simulink library "MOST_Lib"  (R2020b)
settings: Solver=VariableStepAuto  StartTime=0.0  StopTime=10.0  RelTol=1e-3
undefined symbols (not defined in the file): simu, wind, windTurbine, windturbine, X, Y, Z
libraries: nesl_utility x54, sm_lib x50, simulink x4, simulink_extras x1, pid_lib x1, WECSim_Lib_Body_Elements x1
(part 3 of 3)

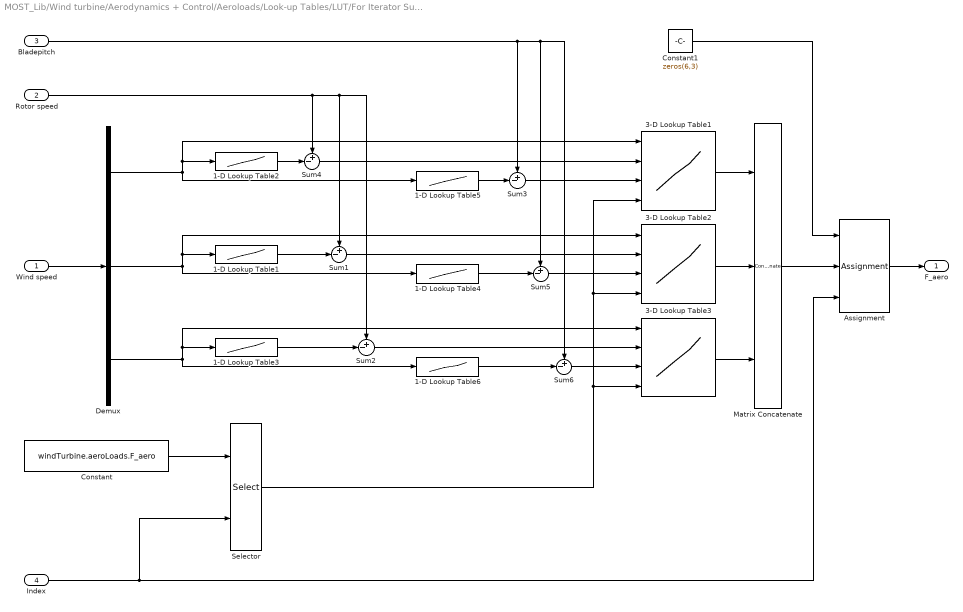
== system MOST_Lib/Wind turbine/Aerodynamics + Control/Aeroloads/Look-up Tables/LUT/For Iterator Subsystem/  ==
  Wind speed : Inport
  Rotor speed : Inport  Port=2
  Bladepitch : Inport  Port=3
  Index : Inport  Port=4
  1-D Lookup Table1 : Lookup_n-D  NumberOfTableDimensions=1  BreakpointsForDimension1=windTurbine.aeroLoads.wind_vec  Table=windTurbine.aeroLoads.omega_vec  InternalRulePriority=Speed  RndMeth=Simplest  InputSameDT=on
  1-D Lookup Table2 : Lookup_n-D  NumberOfTableDimensions=1  BreakpointsForDimension1=windTurbine.aeroLoads.wind_vec  Table=windTurbine.aeroLoads.omega_vec  InternalRulePriority=Speed  RndMeth=Simplest  InputSameDT=on
  1-D Lookup Table3 : Lookup_n-D  NumberOfTableDimensions=1  BreakpointsForDimension1=windTurbine.aeroLoads.wind_vec  Table=windTurbine.aeroLoads.omega_vec  InternalRulePriority=Speed  RndMeth=Simplest  InputSameDT=on
  1-D Lookup Table4 : Lookup_n-D  NumberOfTableDimensions=1  BreakpointsForDimension1=windTurbine.aeroLoads.wind_vec  Table=windTurbine.aeroLoads.bladepitch_vec  InternalRulePriority=Speed  RndMeth=Simplest  InputSameDT=on
  1-D Lookup Table5 : Lookup_n-D  NumberOfTableDimensions=1  BreakpointsForDimension1=windTurbine.aeroLoads.wind_vec  Table=windTurbine.aeroLoads.bladepitch_vec  InternalRulePriority=Speed  RndMeth=Simplest  InputSameDT=on
  1-D Lookup Table6 : Lookup_n-D  NumberOfTableDimensions=1  BreakpointsForDimension1=windTurbine.aeroLoads.wind_vec  Table=windTurbine.aeroLoads.bladepitch_vec  InternalRulePriority=Speed  RndMeth=Simplest  InputSameDT=on
  3-D Lookup Table1 : Lookup_n-D  NumberOfTableDimensions=3  BreakpointsForDimension1=windTurbine.aeroLoads.wind_vec  BreakpointsForDimension2=windTurbine.aeroLoads.omegaerr  BreakpointsForDimension3=windTurbine.aeroLoads.bladepitcherr  TableSource=Input port  Table=squeeze(windturbine.aeroloads.F_aero(:,:,:,1))  ExtrapMethod=Clip  UseLastTableValue=on  InternalRulePriority=Speed  RndMeth=Simplest  InputSameDT=on
      settings: InputPortMap=u0,u1,u2,p221
  3-D Lookup Table2 : Lookup_n-D  NumberOfTableDimensions=3  BreakpointsForDimension1=windTurbine.aeroLoads.wind_vec  BreakpointsForDimension2=windTurbine.aeroLoads.omegaerr  BreakpointsForDimension3=windTurbine.aeroLoads.bladepitcherr  TableSource=Input port  Table=squeeze(windturbine.aeroloads.F_aero(:,:,:,1))  ExtrapMethod=Clip  UseLastTableValue=on  InternalRulePriority=Speed  RndMeth=Simplest  InputSameDT=on
      settings: InputPortMap=u0,u1,u2,p221
  3-D Lookup Table3 : Lookup_n-D  NumberOfTableDimensions=3  BreakpointsForDimension1=windTurbine.aeroLoads.wind_vec  BreakpointsForDimension2=windTurbine.aeroLoads.omegaerr  BreakpointsForDimension3=windTurbine.aeroLoads.bladepitcherr  TableSource=Input port  Table=squeeze(windturbine.aeroloads.F_aero(:,:,:,1))  ExtrapMethod=Clip  UseLastTableValue=on  InternalRulePriority=Speed  RndMeth=Simplest  InputSameDT=on
      settings: InputPortMap=u0,u1,u2,p221
  Assignment : Assignment  NumberOfDimensions=2  DiagnosticForDimensions=Warning  IndexOptions=Index vector (port),Assign all  Indices=1,1  OutputSizes=1,1
  Constant : Constant  Value=windTurbine.aeroLoads.F_aero
  Constant1 : Constant  Value=zeros(6,3)
  Demux : Demux  Outputs=3
  Matrix Concatenate : Concatenate  NumInputs=3  Mode=Multidimensional array  ConcatenateDimension=2
  Selector : Selector  NumberOfDimensions=4  InputPortWidth=3  IndexOptions=Select all,Select all,Select all,Index vector (port)  Indices=[1 3],1,1,1  OutputSizes=1,1,1,1
  Sum{1..6} (6 alike) : Sum  Inputs=+-|
  F_aero : Outport  PortDimensions=[6 3]
  wires:
  Wind speed/1 -> Demux/1
  Demux/3 -> 1-D Lookup Table6/1, 3-D Lookup Table3/1, 1-D Lookup Table3/1
  Demux/2 -> 1-D Lookup Table4/1, 3-D Lookup Table2/1, 1-D Lookup Table1/1
  1-D Lookup Table4/1 -> Sum5/2
  1-D Lookup Table5/1 -> Sum3/2
  1-D Lookup Table6/1 -> Sum6/2
  Sum6/1 -> 3-D Lookup Table3/3
  Sum4/1 -> 3-D Lookup Table1/2
  Sum3/1 -> 3-D Lookup Table1/3
  Demux/1 -> 1-D Lookup Table5/1, 1-D Lookup Table2/1, 3-D Lookup Table1/1
  Sum5/1 -> 3-D Lookup Table2/3
  Sum1/1 -> 3-D Lookup Table2/2
  Sum2/1 -> 3-D Lookup Table3/2
  Rotor speed/1 -> Sum4/1, Sum2/1, Sum1/1
  Constant/1 -> Selector/1
  Index/1 -> Selector/2, Assignment/3
  Selector/1 -> 3-D Lookup Table3/4, 3-D Lookup Table2/4, 3-D Lookup Table1/4
  1-D Lookup Table2/1 -> Sum4/2
  1-D Lookup Table1/1 -> Sum1/2
  1-D Lookup Table3/1 -> Sum2/2
  Bladepitch/1 -> Sum3/1, Sum6/1, Sum5/1
  Assignment/1 -> F_aero/1
  Constant1/1 -> Assignment/1
  3-D Lookup Table1/1 -> Matrix Concatenate/1
  3-D Lookup Table2/1 -> Matrix Concatenate/2
  3-D Lookup Table3/1 -> Matrix Concatenate/3
  Matrix Concatenate/1 -> Assignment/2

== system MOST_Lib/Wind turbine/Aerodynamics + Control/Control/ROSCO/ROSCO controller /Bladepitch control/Integrator with dynamic saturation ==
  omega error : Inport
  minimum pitch : Inport  Port=2
  Constant : Constant  Value=deg2rad(90)
  Gain : Gain  Gain=simu.dt
  Saturation Dynamic : simulink/Discontinuities/Saturation Dynamic  OutMin=[]  OutMax=[]  OutDataTypeStr=Inherit: Same as second input  OutDataType=fixdt(1, 16)  OutScaling=2^-10  DoSatur=off
  Sum : Sum  Inputs=|++
  Unit Delay : UnitDelay  SampleTime=-1  HasFrameUpgradeWarning=on
  integration : Outport
  wires:
  minimum pitch/1 -> Saturation Dynamic/3
  Gain/1 -> Sum/1
  Unit Delay/1 -> Sum/2
  Sum/1 -> Saturation Dynamic/2
  omega error/1 -> Gain/1
  Constant/1 -> Saturation Dynamic/1
  Saturation Dynamic/1 -> Unit Delay/1, integration/1

== matlab function MOST_Lib/Wind turbine/Aerodynamics + Control/Aeroloads/BEM/BEM ==
  data: wind input size=wind.Input.signals.dimensions; q input size=[14 1]; bladepitch input size=1; F_aero_r_bl output size=[6 3]; BEMstruct parameter
function F_aero_r_bl = BEM(wind,q,bladepitch,BEMstruct)

%% INFO

% q: 1-12  -Hub states (no tilt)
%    13    -azimuth
%    14    -rotor omega 

%% CALC AEROLOADS

    pntm=[0 0 0].*BEMstruct.bladedata_r;  
    Cn=0;   Ct=0;    CM=0;
    F_aero_r_bl=zeros(6,3);

           
    R_02hu=Rx(q(4))*Ry(q(5))*Rz(q(6))*BEMstruct.WT_Ry_tilt;
    w_rot_0=q(10:12)+R_02hu*[q(14);0;0];
       
            
    for bl=1:3
        
        R_02bl_root=R_02hu*[1              0                             0             ;
                            0   cos(q(13)+2*pi/3*(bl-1))     -sin(q(13)+2*pi/3*(bl-1)) ;
                            0   sin(q(13)+2*pi/3*(bl-1))      cos(q(13)+2*pi/3*(bl-1))]*BEMstruct.WT_Ry_precone;
        
        a=0;
        at=0;                                                       

        for node=1:length(BEMstruct.bladedata_r)

            
            R_02bl_node=R_02bl_root*[cos(BEMstruct.bladedata_BlCrvAng(node))   0   sin(BEMstruct.bladedata_BlCrvAng(node)) ;
                                                       0                  1                 0                    ;
                                     -sin(BEMstruct.bladedata_BlCrvAng(node))  0   cos(BEMstruct.bladedata_BlCrvAng(node))];


            r_node_0=q(1:3)+R_02bl_root*[BEMstruct.bladedata_BlCrvAC(node);BEMstruct.bladedata_BlSwpAC(node);BEMstruct.bladedata_r(node)];
            v_node_0=q(7:9)+cross(w_rot_0,r_node_0-q(1:3));
           
         
            v_wind_inf_0=[interp3(BEMstruct.WIND_Ydiscr,BEMstruct.WIND_Xdiscr,BEMstruct.WIND_Zdiscr,wind(:,:,:,1),r_node_0(2),r_node_0(1),r_node_0(3));
                          interp3(BEMstruct.WIND_Ydiscr,BEMstruct.WIND_Xdiscr,BEMstruct.WIND_Zdiscr,wind(:,:,:,2),r_node_0(2),r_node_0(1),r_node_0(3));
                          interp3(BEMstruct.WIND_Ydiscr,BEMstruct.WIND_Xdiscr,BEMstruct.WIND_Zdiscr,wind(:,:,:,3),r_node_0(2),r_node_0(1),r_node_0(3))];

            v_wind_rel_bl=R_02bl_node'*(v_wind_inf_0-v_node_0);

            
            VXoverVY=v_wind_rel_bl(1)/v_wind_rel_bl(2);
            s=3*BEMstruct.bladedata_chord(node)/2/pi/BEMstruct.bladedata_r(node);  
            i=1;
            eps=1;

            while eps>BEMstruct.root_tol_rel  &&  i<=BEMstruct.maxit
                phi_i=atan((1-a)/(1+at)*VXoverVY);
                alfa=rad2deg(phi_i-bladepitch)-BEMstruct.bladedata_twist(node);

                CL=interp1(BEMstruct.bladedata_airfoil(:,1,BEMstruct.bladedata_airfoil_index(node)),BEMstruct.bladedata_airfoil(:,2,BEMstruct.bladedata_airfoil_index(node)),alfa);
                CD=interp1(BEMstruct.bladedata_airfoil(:,1,BEMstruct.bladedata_airfoil_index(node)),BEMstruct.bladedata_airfoil(:,3,BEMstruct.bladedata_airfoil_index(node)),alfa);
                CM=interp1(BEMstruct.bladedata_airfoil(:,1,BEMstruct.bladedata_airfoil_index(node)),BEMstruct.bladedata_airfoil(:,4,BEMstruct.bladedata_airfoil_index(node)),alfa);
                Cn=CL*cos(phi_i)+CD*sin(phi_i);
                Ct=CL*sin(phi_i)-CD*cos(phi_i);
               
                Ftip=2/pi*acos(exp(-1.5*(BEMstruct.bladedata_RhubRblade(2)-BEMstruct.bladedata_r(node))/BEMstruct.bladedata_r(node)/abs(sin(phi_i+1e-5)))); % loss tip
                Fhub=2/pi*acos(exp(-1.5*(BEMstruct.bladedata_r(node)-BEMstruct.bladedata_RhubRblade(1))/BEMstruct.bladedata_r(node)/abs(sin(phi_i+1e-5)))); % loss hub
                F=Ftip*Fhub;
               
                k=s*Cn/4/F/sin(phi_i)^2;
                kt=s*Ct/4/F/sin(phi_i)/cos(phi_i);
                if (phi_i>0 && k<=2/3)                
                    a=k/(1+k);                         

                elseif (phi_i>0 && k>2/3)              
                    g1=2*F*k-(10/9-F);
                    g2=2*F*k-F*(4/3-F);
                    g3=2*F*k-(25/9-2*F);
                    a=(g1-sqrt(g2))/g3;                

                elseif (phi_i<0 && k>1)                
                    a=k/(k-1);
                
                elseif (k<=1 && phi_i<0)              
                    a=0;
                end
                
                at=kt/(1-kt);                          

                phi_f=atan((1-a)/(1+at)*VXoverVY);
                i=i+1;
                eps=abs((phi_i-phi_f)/phi_i);

                                
            end
           
           
            if i>BEMstruct.maxit || a==0

                if R(BEMstruct.eps,v_wind_rel_bl(1),bladepitch,q(14),s,node,BEMstruct)*R(pi/2-BEMstruct.eps,v_wind_rel_bl(1),bladepitch,q(14),s,node,BEMstruct)<0
                    phi=Root_find(@(phi)R(phi,v_wind_rel_bl(1),bladepitch,q(14),s,node,BEMstruct),[BEMstruct.eps pi/2],BEMstruct);
                
                elseif Rpb(-pi/4,v_wind_rel_bl(1),bladepitch,q(14),s,node,BEMstruct)*Rpb(-BEMstruct.eps,v_wind_rel_bl(1),bladepitch,q(14),s,node,BEMstruct)<0
                    phi=Root_find(@(phi)Rpb(phi,v_wind_rel_bl(1),bladepitch,q(14),s,node,BEMstruct),[-pi/4 -BEMstruct.eps],BEMstruct);

                else
                    phi=Root_find(@(phi)R(phi,v_wind_rel_bl(1),bladepitch,q(14),s,node,BEMstruct),[pi/2+BEMstruct.eps pi-BEMstruct.eps],BEMstruct);

                end

            alfa=rad2deg(phi-bladepitch)-BEMstruct.bladedata_twist(node);            
            CL=interp1(BEMstruct.bladedata_airfoil(:,1,BEMstruct.bladedata_airfoil_index(node)),BEMstruct.bladedata_airfoil(:,2,BEMstruct.bladedata_airfoil_index(node)),alfa);
            CD=interp1(BEMstruct.bladedata_airfoil(:,1,BEMstruct.bladedata_airfoil_index(node)),BEMstruct.bladedata_airfoil(:,3,BEMstruct.bladedata_airfoil_index(node)),alfa);
            CM=interp1(BEMstruct.bladedata_airfoil(:,1,BEMstruct.bladedata_airfoil_index(node)),BEMstruct.bladedata_airfoil(:,4,BEMstruct.bladedata_airfoil_index(node)),alfa);
            Cn=CL*cos(phi)+CD*sin(phi);
            Ct=CL*sin(phi)-CD*cos(phi);
            Ftip=2/pi*acos(exp(-1.5*(BEMstruct.bladedata_RhubRblade(2)-BEMstruct.bladedata_r(node))/BEMstruct.bladedata_r(node)/abs(sin(phi+1e-5))));
            Fhub=2/pi*acos(exp(-1.5*(BEMstruct.bladedata_r(node)-BEMstruct.bladedata_RhubRblade(1))/BEMstruct.bladedata_r(node)/abs(sin(phi+1e-5))));
            F=Ftip*Fhub;

            kt=s*Ct/4/F/sin(phi)/cos(phi);
            at=kt/(1-kt);
            Vrel2=(v_wind_rel_bl(2)*(1+at)/cos(phi))^2;

            else
            
            Vrel2=(v_wind_rel_bl(1)*(1-a))^2+(v_wind_rel_bl(2)*(1+at))^2;
            
            end
            pntm(node,:)=0.5*BEMstruct.rho_air*BEMstruct.bladedata_chord(node)*Vrel2*[Cn,Ct,CM*BEMstruct.bladedata_chord(node)];        
            

            if anynan([a at])
                a=0; at=0;
            end

        end

        % Remove NaN

        if anynan(pntm)

            temp_y=[[0 0 0];pntm;[0 0 0]];
            temp_x=(1:size(temp_y,1))';
            temp_y=[interp1(temp_x(~isnan(temp_y(:,1))),temp_y(~isnan(temp_y(:,1)),1),temp_x,'linear'),...
                    interp1(temp_x(~isnan(temp_y(:,2))),temp_y(~isnan(temp_y(:,2)),2),temp_x,'linear'),...
                    interp1(temp_x(~isnan(temp_y(:,3))),temp_y(~isnan(temp_y(:,3)),3),temp_x,'linear')];
            pntm=temp_y(2:end-1,:);

        end

        

        F_aero_r_bl(:,bl)=[ (BEMstruct.bladedata_r_int*(pntm(:,1).*cos(BEMstruct.bladedata_BlCrvAng)));
                           -(BEMstruct.bladedata_r_int*pntm(:,2));
                            (BEMstruct.bladedata_r_int*(pntm(:,1).*sin(-BEMstruct.bladedata_BlCrvAng)));
                            (BEMstruct.bladedata_r_int*(pntm(:,2).*(BEMstruct.bladedata_r-BEMstruct.bladedata_RhubRblade(1))*BEMstruct.WT_cos_precone+pntm(:,3).*sin(BEMstruct.bladedata_BlCrvAng)+pntm(:,1).*sin(-BEMstruct.bladedata_BlCrvAng).*BEMstruct.bladedata_BlSwpAC));
                            (BEMstruct.bladedata_r_int*(pntm(:,1).*(BEMstruct.bladedata_r-BEMstruct.bladedata_RhubRblade(1))));
                            (BEMstruct.bladedata_r_int*(pntm(:,3).*cos(BEMstruct.bladedata_BlCrvAng)-pntm(:,1).*cos(BEMstruct.bladedata_BlCrvAng).*BEMstruct.bladedata_BlSwpAC-pntm(:,2).*BEMstruct.bladedata_BlCrvAC))];

        
    end

    

end

%% FUNC

function [root] = Root_find(Fun,Int,BEMstruct)

a = Int(1,1);
b = Int(1,2);
fa = Fun(a);
fb = Fun(b);
it = 0;
s=b;

while abs((b-a)/a)>BEMstruct.root_tol_rel2  &&  it<BEMstruct.maxit2  &&  abs(fb)>BEMstruct.func_tol2

    it = it + 1;
    s = (a + b)/2;
    fs = Fun(s);

    if fa*fs < 0
        b = s;
        fb = fs;
    else
        a = s;
        fa = fs;
    end

end

root = s;

end

% function [root] = Root_find(Fun,Int,ALCS)
% 
% a = Int(1,1);
% b = Int(1,2);
% fa = Fun(a);
% fb = Fun(b);
% fs=fb;
% it = 0;
%                                      
% s=b; c=a;  d=a;    
% mflag = 1;                                
% while abs(b-a)>ALCS.root_tol_rel2 && it<ALCS.maxit2 && abs(fs)>ALCS.func_tol2
%     fc = Fun(c);
%     if fa ~= fc && fb ~=fc                 % inverse quadratic interpolation
%         s = a*fb*fc/((fa - fb)*(fa - fc)) + b*fa*fc/((fb - fa)*(fb - fc))...
%             + c*fa*fb/((fc - fa)*(fc - fb));
%     else                                   % linear interpolation (Secant Method)
%         s = b - fb*(b - a)/(fb - fa);
%     end
%     if (s < min([(3*a + b)/4,b]) || s > max([(3*a + b)/4,b])) || ...
%             (mflag == 1 && abs(s - b) >= abs(b - c)/2) || ...
%             (mflag == 0 && abs(s - b) >= abs(c - d)/2) || ...
%             (mflag == 1 && abs(b - c) < ALCS.root_tol_rel2) || ...
%             (mflag == 0 && abs(c - d) < ALCS.root_tol_rel2)
%         s = (a + b)/2;
%         mflag = 1;
%     else
%         mflag = 0;
%     end
%     it = it + 1;
%     fs = Fun(s);
%         
%     if fa*fs < 0
%         d = c;                             % if c was b_{k - 1}, d would be b_{k - 2}
%         c = b;
%         b = s;
%         fb = fs;
%     else
%         a = s;
%         fa = fs;
%     end
%     
% end
% 
% root = s;
% 
% end

function resR=R(phi,U_inf,blpitch,omega,solidity,node,BEMstruct)


alfa=rad2deg(phi-blpitch)-BEMstruct.bladedata_twist(node);

CL=interp1(BEMstruct.bladedata_airfoil(:,1,BEMstruct.bladedata_airfoil_index(node)),BEMstruct.bladedata_airfoil(:,2,BEMstruct.bladedata_airfoil_index(node)),alfa);
CD=interp1(BEMstruct.bladedata_airfoil(:,1,BEMstruct.bladedata_airfoil_index(node)),BEMstruct.bladedata_airfoil(:,3,BEMstruct.bladedata_airfoil_index(node)),alfa);

Cn=CL*cos(phi)+CD*sin(phi);
Ct=CL*sin(phi)-CD*cos(phi);

Ftip=2/pi*acos(exp(-1.5*(BEMstruct.bladedata_RhubRblade(2)-BEMstruct.bladedata_r(node))/BEMstruct.bladedata_r(node)/abs(sin(phi+1e-5)))); 
Fhub=2/pi*acos(exp(-1.5*(BEMstruct.bladedata_r(node)-BEMstruct.bladedata_RhubRblade(1))/BEMstruct.bladedata_r(node)/abs(sin(phi+1e-5)))); 
F=Ftip*Fhub;

k=solidity*Cn/4/F/sin(phi)^2;
kt=solidity*Ct/4/F/sin(phi)/cos(phi);

if  k<=2/3                
    a=k/(1+k);                         

else
    g1=2*F*k-(10/9-F);
    g2=2*F*k-F*(4/3-F);
    g3=2*F*k-(25/9-2*F)+1e-6;
    a=(g1-sqrt(g2))/g3;                

end

at=kt/(1-kt);                          

resR=sin(phi)/(1-a)-cos(phi)/(omega*BEMstruct.bladedata_r(node)/U_inf*(1+at));


end

function resRpb=Rpb(phi,U_inf,blpitch,omega,solidity,node,BEMstruct)

alfa=rad2deg(phi-blpitch)-BEMstruct.bladedata_twist(node);

CL=interp1(BEMstruct.bladedata_airfoil(:,1,BEMstruct.bladedata_airfoil_index(node)),BEMstruct.bladedata_airfoil(:,2,BEMstruct.bladedata_airfoil_index(node)),alfa);
CD=interp1(BEMstruct.bladedata_airfoil(:,1,BEMstruct.bladedata_airfoil_index(node)),BEMstruct.bladedata_airfoil(:,3,BEMstruct.bladedata_airfoil_index(node)),alfa);

Cn=CL*cos(phi)+CD*sin(phi);
Ct=CL*sin(phi)-CD*cos(phi);

Ftip=2/pi*acos(exp(-1.5*(BEMstruct.bladedata_RhubRblade(2)-BEMstruct.bladedata_r(node))/BEMstruct.bladedata_r(node)/abs(sin(phi+1e-5)))); 
Fhub=2/pi*acos(exp(-1.5*(BEMstruct.bladedata_r(node)-BEMstruct.bladedata_RhubRblade(1))/BEMstruct.bladedata_r(node)/abs(sin(phi+1e-5)))); 
F=Ftip*Fhub;

k=solidity*Cn/4/F/sin(phi)^2;
kt=solidity*Ct/4/F/sin(phi)/cos(phi);
                       
resRpb=sin(phi)*(1-k)-cos(phi)/(omega*BEMstruct.bladedata_r(node)/U_inf)*(1-kt);


end


function [Rx] = Rx(phi)

        Rx=[1      0             0   ;
            0   cos(phi)    -sin(phi);
            0   sin(phi)    cos(phi)]; 
end

function [Ry] = Ry(theta)

       Ry=[cos(theta)   0   sin(theta);
               0        1       0;
           -sin(theta)  0   cos(theta)]; 
end

function [Rz] = Rz(psi)

       Rz=[cos(psi)  -sin(psi)  0;
           sin(psi)  cos(psi)   0;
              0          0      1];

end

== matlab function MOST_Lib/Wind turbine/Aerodynamics + Control/Aeroloads/Look-up Tables/Relative Wind/Calc Relative Wind ==
  data: wind input size=wind.Input.signals.dimensions; q input size=[14 1]; v_wind_rel_bl_x output size=[3 1]; tilt input; precone input; bladeDiscr input; BlCrvAC input; BlSwpAC input; BlCrvAng input; Wind_Xdiscr input; Wind_Ydiscr input; Wind_Zdiscr input
function v_wind_rel_bl_x = Calc_relative_wind(wind, q, tilt, precone, bladeDiscr, BlCrvAC, BlSwpAC, BlCrvAng, Wind_Xdiscr, Wind_Ydiscr, Wind_Zdiscr)

%% INFO

% q: 1-12  -Hub states (no tilt)
%    13    -azimuth
%    14    -rotor omega 

%% MAIN
v_wind_rel_bl_x=zeros(3,1);

R_02hu=Rx(q(4))*Ry(q(5))*Rz(q(6))*Ry(tilt);
    w_rot_0=q(10:12)+R_02hu*[q(14);0;0];


for bl=1:3

    R_02bl_root=R_02hu*[1              0                             0             ;
                        0   cos(q(13)+2*pi/3*(bl-1))     -sin(q(13)+2*pi/3*(bl-1)) ;
                        0   sin(q(13)+2*pi/3*(bl-1))      cos(q(13)+2*pi/3*(bl-1))]*Ry(precone);
    
    
    for node=1:length(bladeDiscr)

        R_02bl_node=R_02bl_root*[cos(BlCrvAng(node))   0   sin(BlCrvAng(node)) ;
                                         0             1            0          ;
                                 -sin(BlCrvAng(node))  0   cos(BlCrvAng(node))];


        r_node_0=q(1:3)+R_02bl_root*[BlCrvAC(node);BlSwpAC(node);bladeDiscr(node)];
        v_node_0=q(7:9)+cross(w_rot_0,r_node_0-q(1:3));


        v_wind_inf_0=[interp3(Wind_Ydiscr,Wind_Xdiscr,Wind_Zdiscr,wind(:,:,:,1),r_node_0(2),r_node_0(1),r_node_0(3));
                      interp3(Wind_Ydiscr,Wind_Xdiscr,Wind_Zdiscr,wind(:,:,:,2),r_node_0(2),r_node_0(1),r_node_0(3));
                      interp3(Wind_Ydiscr,Wind_Xdiscr,Wind_Zdiscr,wind(:,:,:,3),r_node_0(2),r_node_0(1),r_node_0(3))];


        v_wind_rel_bl_x(bl,1)=v_wind_rel_bl_x(bl,1)+R_02bl_node(:,1)'*(v_wind_inf_0-v_node_0);

    end    

    v_wind_rel_bl_x(bl,1)=v_wind_rel_bl_x(bl,1)/length(bladeDiscr);

end
end
%% FUNCTIONS
function [Rx] = Rx(phi)

        Rx=[1      0             0   ;
            0   cos(phi)    -sin(phi);
            0   sin(phi)    cos(phi)]; 
end

function [Ry] = Ry(theta)

       Ry=[cos(theta)   0   sin(theta);
               0        1       0;
           -sin(theta)  0   cos(theta)]; 
end

function [Rz] = Rz(psi)

       Rz=[cos(psi)  -sin(psi)  0;
           sin(psi)  cos(psi)   0;
              0          0      1];

end
